simulink model "jiasuduji"  (R2017b)
settings: Solver=VariableStepAuto  StartTime=0.0  StopTime=10.0  RelTol=1e-3
libraries: sharedtransform x1
settings Model: Creator=chenshiming  LastModifiedBy=chenshiming

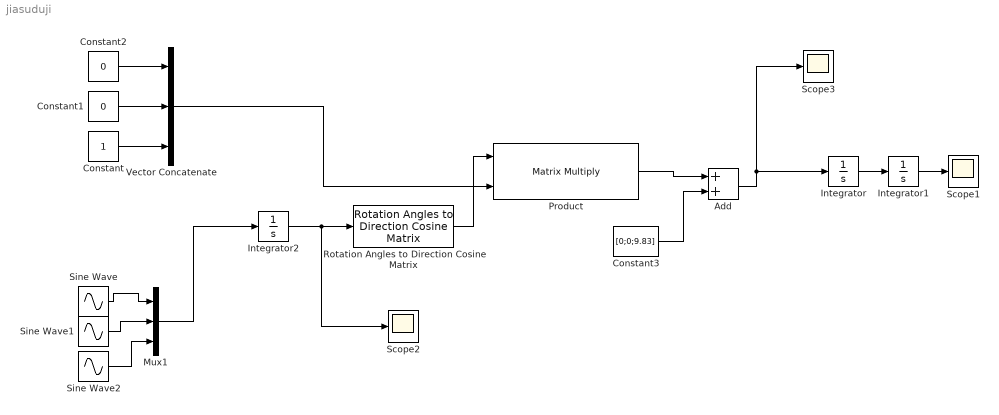
== system jiasuduji ==
  Add : Sum
  Constant : Constant
  Constant1 : Constant  Value=0
  Constant2 : Constant  Value=0
  Constant3 : Constant  Value=[0;0;9.83]
  Integrator : Integrator
  Integrator1 : Integrator
  Integrator2 : Integrator
  Mux1 : Mux  Inputs=3
  Product : Product  Multiplication=Matrix(*)
  Rotation Angles to Direction Cosine Matrix : sharedtransform/Rotation Angles to Direction Cosine Matrix  rotationOrder=ZYX
      settings: SourceProductBaseCode=AE
  Scope1 : Scope
  Scope2 : Scope
  Scope3 : Scope
  Sine Wave : Sin  Amplitude=0.1  SampleTime=0
  Sine Wave1 : Sin  Amplitude=0.2  SampleTime=0
  Sine Wave2 : Sin  Amplitude=0.2  SampleTime=0
  Vector Concatenate : Concatenate  NumInputs=3
  wires:
  Constant/1 -> Vector Concatenate/3
  Constant2/1 -> Vector Concatenate/1
  Constant1/1 -> Vector Concatenate/2
  Integrator/1 -> Integrator1/1
  Sine Wave/1 -> Mux1/1
  Integrator1/1 -> Scope1/1
  Integrator2/1 -> Scope2/1, Rotation Angles to Direction Cosine Matrix/1
  Sine Wave1/1 -> Mux1/2
  Sine Wave2/1 -> Mux1/3
  Mux1/1 -> Integrator2/1
  Rotation Angles to Direction Cosine Matrix/1 -> Product/1
  Vector Concatenate/1 -> Product/2
  Product/1 -> Add/1
  Add/1 -> Integrator/1, Scope3/1
  Constant3/1 -> Add/2
